simulink model "HW01_Single_SMD"  (R2022b)
settings: Solver=VariableStepAuto  StartTime=0.0  StopTime=10.0  RelTol=1e-3
libraries: simulink x1
settings Model: Creator=bojack  LastModifiedBy=bojack

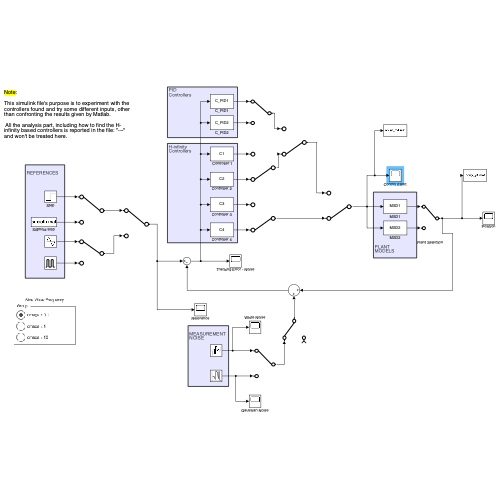
[thumbnail: Simulink's stored preview of the top-level diagram]
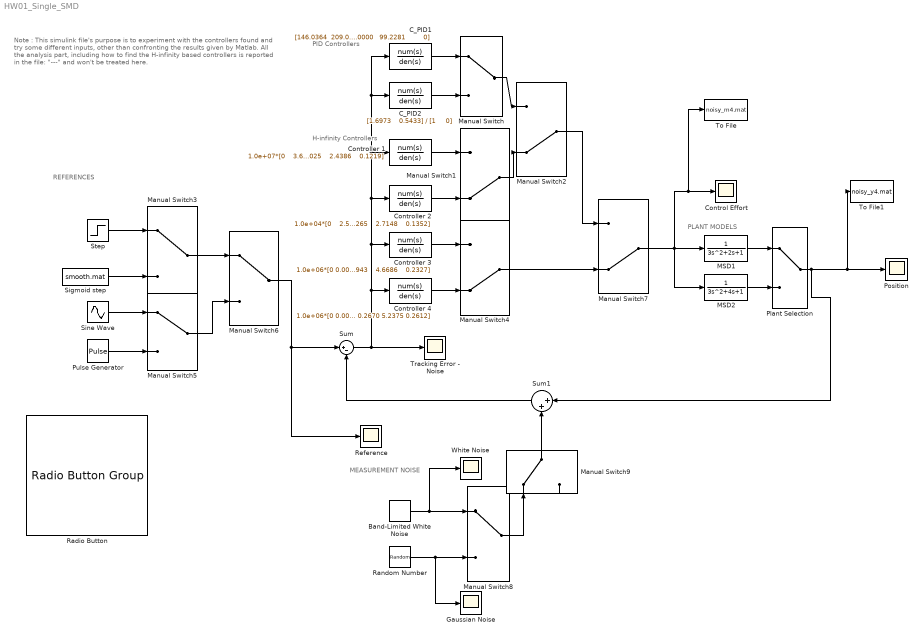
== system HW01_Single_SMD ==
  note: Note :
      |
      | This simulink file's purpose is to experiment with the controllers found and try some different inputs, other than confronting the results given by Matlab.
      |
      | All the analysis part, including how to find the H-infinity based controllers is reported in the file: "---" and won't be treated here.
  note: PLANT
      | MODELS
  note: MEASUREMENT
      | NOISE
  note: REFERENCES
  note: PID
      | Controllers
  note: H-infinity
      | Controllers
  " Controller 1" : TransferFcn  Numerator="1.0e+07*[0    3.6384    2.4256    1.2128]"  Denominator="1.0e+06* [0.0000    0.0025    2.4386    0.1219]"
      mask Display: disp('C1');
  Band-Limited White Noise : simulink/Sources/Band-Limited White Noise  Cov=[0.000005]  Ts=0.01  seed=[23341]
  C_PID1 : TransferFcn  Numerator="[146.0364  209.0861   74.8100]"  Denominator="[1.0000   99.2281         0]"
      mask Display: disp('C_PID1');
  C_PID2 : TransferFcn  Numerator="[1.6973    0.5433]"  Denominator="[1     0]"
      mask Display: disp('C_PID2');
  Control Effort : Scope
  Controller 2 : TransferFcn  Numerator="1.0e+04*[0    2.5678    1.7119    0.8559]"  Denominator="1.0e+03*[0.0010    0.2265    2.7148    0.1352]"
      mask Display: disp('C2');
  Controller 3 : TransferFcn  Numerator=1.0e+06*[0 0.0000 5.0358 3.3572 1.6786]  Denominator="1.0e+05 *[0.0000 0.0059  0.2943    4.6686    0.2327]"
      mask Display: disp('C3');
  Controller 4 : TransferFcn  Numerator=1.0e+06*[0 0.0000 5.0847 3.3898 1.6949]  Denominator=1.0e+05*[0.0000 0.0041 0.2670 5.2375 0.2612]
      mask Display: disp('C4');
  Gaussian Noise : Scope
  MSD1 : TransferFcn  Denominator=[3 2 1]
      mask Display: disp('MSD1');
  MSD2 : TransferFcn  Denominator=[3 4 1]
      mask Display: disp('MSD2');
  Manual Switch{,3,5..6,8..9} (6 alike) : ManualSwitch
  Manual Switch{1..2,4,7} (4 alike) : ManualSwitch  CurrentSetting=0
  Plant Selection : ManualSwitch
  Position : Scope
  Pulse Generator : DiscretePulseGenerator  PulseType=Time based  Period=3  PulseWidth=50
  Radio Button : RadioButtonGroup  SelectedLabel=omega = 0.1  ButtonGroupName=Group
      settings: Values={{'omega = 0.1', 'omega = 1', 'omega = 10'}, [0.1 1 10]}
  Random Number : RandomNumber  Variance=0.001  SampleTime=0.01
  Reference : Scope
  Sigmoid step : FromFile  FileName=smooth.mat  OutDataTypeStr=double  SampleTime=0.01
  Sine Wave : Sin  Frequency=0.1  SampleTime=0
  Step : Step  Time=0  SampleTime=0
  Sum : Sum  Inputs=|+-
  Sum1 : Sum  Inputs=|++
  To File : ToFile  Filename=noisy_m4.mat  MatrixName=u_n4  SampleTime=0.01
  To File1 : ToFile  Filename=noisy_y4.mat  MatrixName=y_n4  SampleTime=0.01
  Tracking Error - Noise : Scope
  White Noise : Scope
  wires:
  Sum/1 -> Tracking Error - Noise/1, Controller 4/1, Controller 2/1, " Controller 1"/1, C_PID2/1, C_PID1/1, Controller 3/1
  Step/1 -> Manual Switch3/1
  Sigmoid step/1 -> Manual Switch3/2
  Sine Wave/1 -> Manual Switch5/1
  Manual Switch3/1 -> Manual Switch6/1
  Manual Switch5/1 -> Manual Switch6/2
  Manual Switch6/1 -> Reference/1, Sum/1
  Band-Limited White Noise/1 -> Manual Switch8/1, White Noise/1
  Sum1/1 -> Sum/2
  Random Number/1 -> Gaussian Noise/1, Manual Switch8/2
  MSD2/1 -> Plant Selection/2
  MSD1/1 -> Plant Selection/1
  C_PID2/1 -> Manual Switch/2
  C_PID1/1 -> Manual Switch/1
  " Controller 1"/1 -> Manual Switch1/1
  Controller 2/1 -> Manual Switch1/2
  Controller 3/1 -> Manual Switch4/1
  Controller 4/1 -> Manual Switch4/2
  Manual Switch/1 -> Manual Switch2/1
  Manual Switch1/1 -> Manual Switch2/2
  Manual Switch4/1 -> Manual Switch7/2
  Manual Switch2/1 -> Manual Switch7/1
  Manual Switch7/1 -> MSD1/1, MSD2/1, To File/1, Control Effort/1
  Plant Selection/1 -> Sum1/1, To File1/1, Position/1
  Manual Switch9/1 -> Sum1/2
  Manual Switch8/1 -> Manual Switch9/1
  Pulse Generator/1 -> Manual Switch5/2
